simulink model "populationDynamics"  (R2018a)
settings: Solver=FixedStepDiscrete  StartTime=0.0  StopTime=100  RelTol=1e-3  EnableMultiTasking=on
PreLoadFcn:
  | P0 = 1e5;  % Initial Population
  | L = 1e6;    % Carrying Capacity
  | r = 1.5e-6;    % Reproduction Rate
settings Model: Creator=nicholas  LastModifiedBy=bneiswan
settings DataIOCC: SaveFormat=Array  SaveTime=off  SignalLoggingName=logsOut
settings OptimizationCC: BlockReduction=off  BooleanDataType=off  ExpressionDepthLimit=2147483647  InitFltsAndDblsToZero=on  LifeSpan=inf
settings DebuggingCC: SaveWithParameterizedLinksMsg=none  UnderspecifiedInitializationDetection=Classic  MergeDetectMultiDrivingBlocksExec=none  CheckExecutionContextPreStartOutputMsg=on  CheckExecutionContextRuntimeOutputMsg=on  SignalResolutionControl=TryResolveAllWithWarning  MultiTaskDSMMsg=warning  MultiTaskCondExecSysMsg=none  ParameterPrecisionLossMsg=none  FcnCallInpInsideContextMsg=warning  AllowSymbolicDim=off  StateNameClashWarn=warning  SFUnexpectedBacktrackingDiag=warning  SFNoUnconditionalDefaultTransitionDiag=warning  SFExecutionAtInitializationDiag=none
settings HardwareCC: ProdBitPerPointer=32  ProdBitPerSizeT=32  ProdBitPerPtrDiffT=32  ProdLargestAtomicFloat=None  ProdIntDivRoundTo=Undefined  ProdEndianess=Unspecified  ProdWordSize=32  ProdHWDeviceType=32-bit Generic  TargetUnknown=on
settings ModelReferenceCC: PropagateSignalLabelsOutOfModel=off
settings CodeAppCC: StateflowObjectComments=on
settings GRTTargetCC: TargetFcnLib=ansi_tfl_tmw.mat  TargetLangStandard=C89/C90 (ANSI)  GeneratePreprocessorConditionals=Disable all  CombineOutputUpdateFcns=off  GRTInterface=on
settings ConfigComp: CovMetricSettings=dw  CovHtmlReporting=on  CovSaveCumulativeToWorkspaceVar=on  CovSaveSingleToWorkspaceVar=on  CovExternalEMLEnable=off  CovSFcnEnable=off

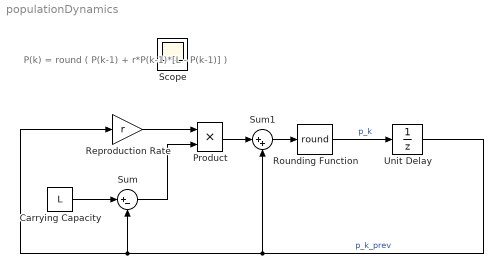
== system populationDynamics ==
  note: P(k) = round ( P(k-1) + r*P(k-1)*[L - P(k-1)] )
  Carrying Capacity : Constant  Value=L
  Product : Product  RndMeth=Zero
  Reproduction Rate : Gain  Gain=r
  Rounding Function : Rounding  Operator=round
  Sum : Sum  Inputs=|+-
  Sum1 : Sum  Inputs=|++
  Unit Delay : UnitDelay  InitialCondition=P0
      settings: AttributesFormatString=Sample Time = %<SampleTime>\nInitial Cond = %<X0>
  Scope : Scope
  wires:
  Sum/1 -> Product/2
  Unit Delay/1 -> Reproduction Rate/1, Sum/2, Sum1/2  "p_k_prev"
  Carrying Capacity/1 -> Sum/1
  Product/1 -> Sum1/1
  Reproduction Rate/1 -> Product/1
  Rounding Function/1 -> Unit Delay/1  "p_k"
  Sum1/1 -> Rounding Function/1
